simulink model "Ex9_10model"  (R2013a)
settings: Solver=ode45  StartTime=0.0  StopTime=3  RelTol=1e-3
settings Model: Creator=JLS  LastModifiedBy=John
settings DataIOCC: SignalLoggingSaveFormat=ModelDataLogs
settings OptimizationCC: ExpressionDepthLimit=2147483647
settings DebuggingCC: FcnCallInpInsideContextMsg=UseLocalSettings
settings GRTTargetCC: CombineOutputUpdateFcns=off  GRTInterface=on

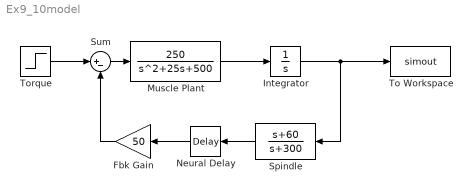
== system Ex9_10model ==
  Fbk Gain : Gain  Gain=50
  Integrator : Integrator
  Muscle Plant : TransferFcn  Numerator=250  Denominator=[1 25 500]
  Neural Delay : TransportDelay  DelayTime=.03
  Spindle : TransferFcn  Numerator=[1 60]  Denominator=[1 300]
  Sum : Sum  Inputs=|+-
  To Workspace : ToWorkspace  VariableName=simout  SampleTime=-1
  Torque : Step  Time=0  After=5  SampleTime=0
  wires:
  Sum/1 -> Muscle Plant/1
  Muscle Plant/1 -> Integrator/1
  Integrator/1 -> To Workspace/1, Spindle/1
  Fbk Gain/1 -> Sum/2
  Torque/1 -> Sum/1
  Neural Delay/1 -> Fbk Gain/1
  Spindle/1 -> Neural Delay/1
